simulink model "eq_mouvement"  (R2024b)
settings: Solver=FixedStepAuto  StartTime=0.0  StopTime=10.0  FixedStep=Ts  RelTol=1e-3
settings Model: Creator=marti  LastModifiedBy=marti

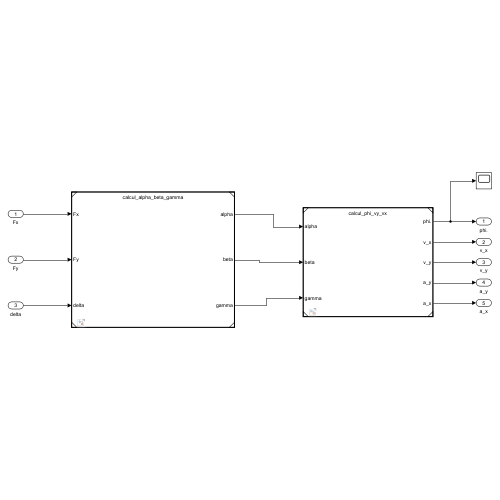
[thumbnail: Simulink's stored preview of the top-level diagram]
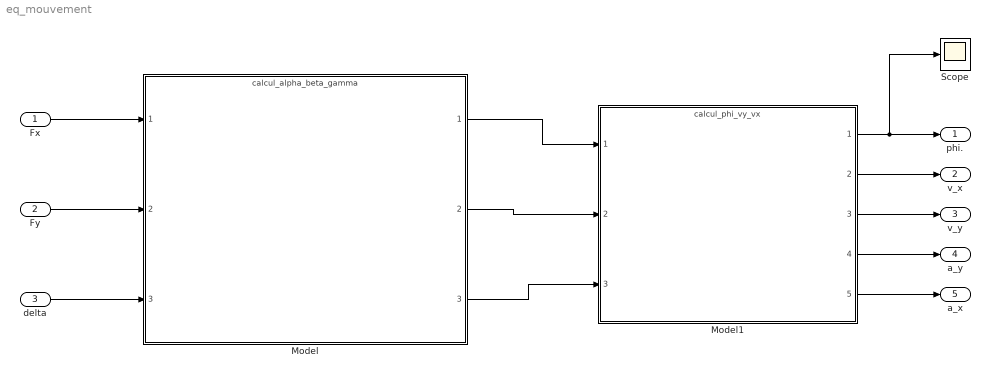
== system eq_mouvement ==
  Fx : Inport
  Fy : Inport  Port=2
  delta : Inport  Port=3
  Model : ModelReference  ModelNameDialog=calcul_alpha_beta_gamma.slx  SimulationMode=Normal  ModelReferenceVersion=1.4
  Model1 : ModelReference  ModelNameDialog=calcul_phi_vy_vx.slx  SimulationMode=Normal  ModelReferenceVersion=1.16
  Scope : Scope
  phi. : Outport
  v_x : Outport  Port=2
  v_y : Outport  Port=3
  a_y : Outport  Port=4
  a_x : Outport  Port=5
  wires:
  Model/1 -> Model1/1
  Model/2 -> Model1/2
  Model/3 -> Model1/3
  Fx/1 -> Model/1
  Fy/1 -> Model/2
  delta/1 -> Model/3
  Model1/1 -> Scope/1, phi./1
  Model1/2 -> v_x/1
  Model1/3 -> v_y/1
  Model1/4 -> a_y/1
  Model1/5 -> a_x/1
